simulink model "klima"  (R2020a)
settings: Solver=VariableStepAuto  StartTime=0.0  StopTime=60  MaxStep=0.01  RelTol=1e-3
settings Model: Creator=muham  LastModifiedBy=muham

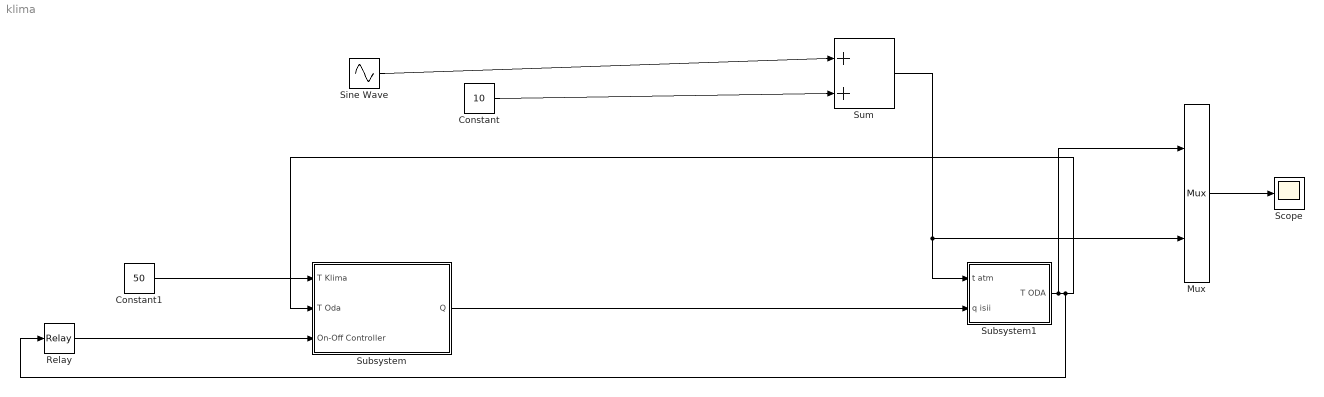
== system klima ==
  Constant : Constant  Value=10
  Constant1 : Constant  Value=50
  Mux : Mux  Inputs=2
  Relay : Relay  OnSwitchValue=24  OffSwitchValue=20  OnOutputValue=0  OffOutputValue=1
  Scope : Scope
  Sine Wave : Sin  Amplitude=15  SampleTime=0
  Subsystem : Subsystem
  Subsystem1 : Subsystem
  Sum : Sum  Inputs=|++
  wires:
  Subsystem/1(Q) -> Subsystem1/2(q isii)
  Constant/1 -> Sum/2
  Sine Wave/1 -> Sum/1
  Sum/1 -> Mux/2, Subsystem1/1(t atm)
  Constant1/1 -> Subsystem/1(T Klima)
  Relay/1 -> Subsystem/3(On-Off Controller)
  Subsystem1/1(T ODA) -> Mux/1, Relay/1, Subsystem/2(T Oda)
  Mux/1 -> Scope/1

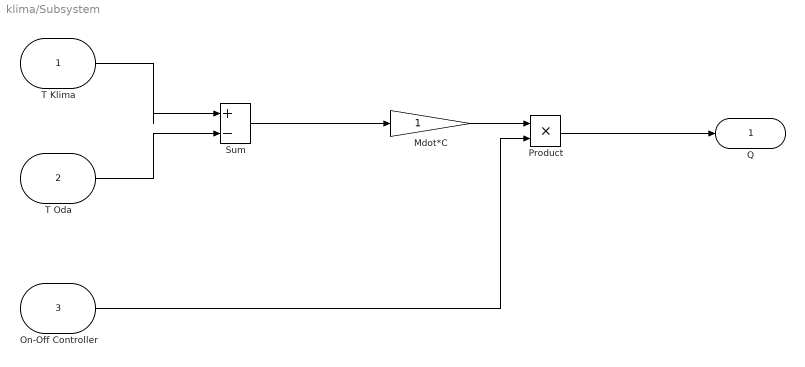
== system klima/Subsystem ==
  T Klima : Inport
  T Oda : Inport  Port=2
  On-Off Controller : Inport  Port=3
  Mdot*C : Gain
  Product : Product
  Sum : Sum  Inputs=|+-
  Q : Outport
  wires:
  On-Off Controller/1 -> Product/2
  T Oda/1 -> Sum/2
  Mdot*C/1 -> Product/1
  Product/1 -> Q/1
  T Klima/1 -> Sum/1
  Sum/1 -> Mdot*C/1

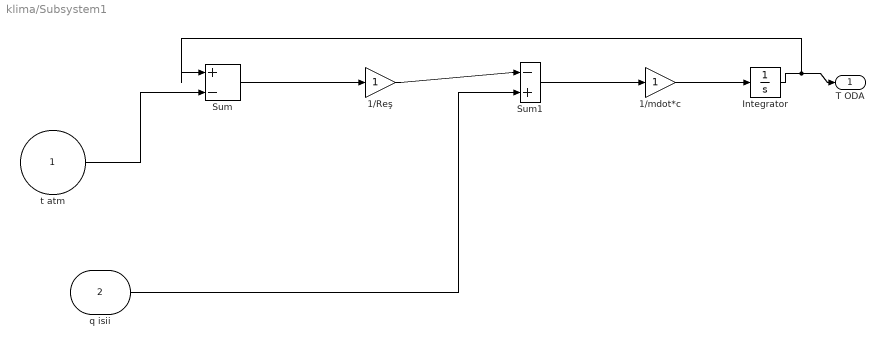
== system klima/Subsystem1 ==
  t atm : Inport
  q isii : Inport  Port=2
  1/Reş : Gain
  1/mdot*c : Gain
  Integrator : Integrator
  Sum : Sum  Inputs=|+-
  Sum1 : Sum  Inputs=|-+
  T ODA : Outport
  wires:
  t atm/1 -> Sum/2
  1/Reş/1 -> Sum1/1
  1/mdot*c/1 -> Integrator/1
  Sum1/1 -> 1/mdot*c/1
  q isii/1 -> Sum1/2
  Sum/1 -> 1/Reş/1
  Integrator/1 -> Sum/1, T ODA/1
